simulink model "commander"  (R2021a)
settings: Solver=FixedStepAuto  StartTime=0.0  StopTime=5  FixedStep=0.02  RelTol=1e-3
(part 2 of 2)

== stateflow chart commander/Commander ==
  state initialize [parallel]
    en:
    % 初始化结构体（全局变量结尾加下划线）
    vehicle_status_out_ = px4_vehicle_status_zero();
    led_control_out_ = px4_led_control_zero();
    armed_out_ = px4_actuator_armed_zero();
    home_position_out_ = px4_home_position_zero();
    vehicle_status_flags_out_ = px4_vehicle_status_flags_zero();
    land_detector_ = land_detector;
    battery_status_out_ = px4_battery_status_zero();
    internal_state_out_ = px4_commander_state_zero();
    % 初始化相关的结构体成员变量
    land_detector_.landed = true;
    % XXX for now just set sensors as initialized
    vehicle_status_flags_out_.condition_system_sensors_initialized = true;
    % We want to accept RC inputs as default
    vehicle_status_out_.rc_input_mode = uint8(PX4_VEHICLE_STATUS.RC_IN_MODE_DEFAULT);
    vehicle_status_out_.nav_state = uint8(PX4_VEHICLE_STATUS.NAVIGATION_STATE_MANUAL);
    vehicle_status_out_.nav_state_timestamp = uint64(getSimulationTime * 1e+6);
    vehicle_status_out_.arming_state = uint8(PX4_VEHICLE_STATUS.ARMING_STATE_INIT);
    % mark all signals lost as long as they haven't been found
    vehicle_status_out_.rc_signal_lost = true;
    vehicle_status_out_.data_link_lost = true;
    % vehicle_status_flags
    vehicle_status_flags_out_.offboard_control_signal_lost = true;
    vehicle_status_flags_out_.condition_power_input_valid = true;
    vehicle_status_flags_out_.rc_calibration_valid = true;
    % default for vtol is rotary wing
    vtol_status_.vtol_in_rw_mode = true;
    % LED和蜂鸣器初始化
    led_init();
    buzzer_init();
    % 参数更新
    get_circuit_breaker_params();
    % 更新载具类型
    update_vehicle_status();
    % 记录commander启动时间
    boot_timestamp_ = uint64(getSimulationTime * 1e+6);
    % 初始化相关时间
    last_lpos_fail_time_us_ = boot_timestamp_;
    last_gpos_fail_time_us_ = boot_timestamp_;
    last_lvel_fail_time_us_ = boot_timestamp_;
    % 解锁方式
    arm_auth_init();
    settings: executionOrder=1
  state topic_update [parallel]
    settings: executionOrder=2
    state parameters_update [parallel]
      en,du:
      % 是否使能避障
      vehicle_status_flags_out_.avoidance_system_required = boolean(COM_OBS_AVOID);
      % 参数更新
      if (hasChanged(params_update.timestamp) || param_init_forced_)
      % updateParams();
      % 未解锁状态下才能修改的参数
      if(~actuator_armed.armed)
      is_rotary = is_rotary_wing(vehicle_status_out_) || (is_vtol(vehicle_status_out_) && vtol_status.vtol_in_rw_mode);
      is_fixed = is_fixed_wing(vehicle_status_out_) ||  (is_vtol(vehicle_status_out_) && ~vtol_status.vtol_in_rw_mode);
      is_ground = is_ground_rover(vehicle_status_out_);
      end
      % 飞机模式优先级高于手动
      if (is_rotary)
      vehicle_status_out_.vehicle_type = uint8(PX4_VEHICLE_STATUS.VEHICLE_TYPE_ROTARY_WING);
      elseif (is_fixed)
      vehicle_status_out_.vehicle_type = uint8(PX4_VEHICLE_STATUS.VEHICLE_TYPE_FIXED_WING);
      elseif (is_ground)
      vehicle_status_out_.vehicle_type = uint8(PX4_VEHICLE_STATUS.VEHICLE_TYPE_ROVER);
      end
      vehicle_status_out_.is_vtol = is_vtol(vehicle_status_out_);
      vehicle_status_out_.is_vtol_tailsitter = is_vtol_tailsitter(vehicle_status_out_);
      % check and update system / component ID
      vehicle_status_out_.system_id = MAV_SYS_ID;
      vehicle_status_out_.component_id = MAV_COMP_ID;
      initialize.get_circuit_breaker_params();
      status_changed_ = true;
      % 不受解锁状态影响就可以修改的参数
      vehicle_status_flags_out_.avoidance_system_required = boolean(COM_OBS_AVOID);
      vehicle_status_out_.rc_input_mode = uint8(COM_RC_IN_MODE);
      % 解锁条件
      arm_requirements_.arm_authorization = boolean(COM_ARM_AUTH_REQ);
      arm_requirements_.esc_check = boolean(COM_ARM_CHK_ESCS);
      arm_requirements_.global_position = ~COM_ARM_WO_GPS;
      arm_requirements_.mission = boolean(COM_ARM_MIS_REQ);
      arm_requirements_.geofence = (GF_ACTION > PX4_GEOFENCE_RESULT.GF_ACTION_NONE);
      % 飞行模式槽
      flight_mode_slots_(1) = COM_FLTMODE1;
      flight_mode_slots_(2) = COM_FLTMODE2;
      flight_mode_slots_(3) = COM_FLTMODE3;
      flight_mode_slots_(4) = COM_FLTMODE4;
      flight_mode_slots_(5) = COM_FLTMODE5;
      flight_mode_slots_(6) = COM_FLTMODE6;
      % 检查airmode：yaw airmode需要使用解锁开关
      if ((MC_AIRMODE~= PARAM_INVALID) && (RC_MAP_ARM_SW ~= PARAM_INVALID))
      if (MC_AIRMODE == 2) && (RC_MAP_ARM_SW == 0)
      % airmode = 1; % change to roll/pitch airmode
      % param_set(param_airmode, &airmode);
      sprintf("Yaw Airmode requires the use of an Arm Switch")
      end
      param_init_forced_ = false;
      end
      end
      settings: executionOrder=1
    state offboard_control [parallel]
      en,du:
      % 预留
      settings: executionOrder=2
    state power_update [parallel]
      settings: executionOrder=3
      (default) -> (junction 288)
      power_update -> (junction 288) : [hasChanged(system_power.timestamp) && ...
          | (uint64(getSimulationTime * 1e+6) - system_power.timestamp) < 1e+6]
      (junction 288) -> (junction 289) [order 1] : [system_power.servo_valid && ...
          | ~system_power.brick_valid && ...
          | ~system_power.usb_connected]
      (junction 288) -> (junction 290) [order 2] : {vehicle_status_flags_out_.condition_power_input_valid = true;}
      (junction 289) -> (junction 291) : % 在只有舵机电源有效的情况下飞行，这是不安全的
          | {vehicle_status_flags_out_.condition_power_input_valid = false;}
      (junction 291) -> (junction 290)
      (junction 290) -> (junction 292)
    state land_detector_auto_disarm_update [parallel]
      en,du:
      if (hasChanged(land_detector.timestamp) && actuator_armed.armed)
      if ( ~home_position.manual_home && ...
      (should_set_home_on_takeoff_ == true) && land_detector_.landed && ...
      (uint64(getSimulationTime * 1e+6) > INAIR_RESTART_HOLDOFF_INTERVAL))
      if (was_landed)
      should_set_home_on_takeoff_ = ~set_home_position();
      elseif (COM_HOME_IN_AIR)
      should_set_home_on_takeoff_ = ~set_in_air_home_position();
      end
      end
      end
      % Auto disarm after 5 seconds if kill switch is engaged
      if (actuator_armed.armed && (actuator_armed.manual_lockdown || actuator_armed.lockdown))
      if (elapsed(sec) > COM_KILL_DISARM && actuator_armed.manual_lockdown)
      send(EVT_KILL_SWITCH, arming_state_transition);
      elseif (elapsed(sec) > COM_KILL_DISARM)
      send(EVT_LOCKDOWN, arming_state_transition);
      end
      end
      settings: executionOrder=4
      state land
        en:
        if (uint64(getSimulationTime) ~= 0)
        sprintf("mavlink_log_info: Landing detected")
        end
        vehicle_status_out_.takeoff_time = uint64(0);
        was_landed = land_detector.landed;
        du:
        % 在地面期间，有以下两种情况会自动上锁
        % situation1. 着陆后，经过COM_DISARM_LAND秒后，无人机自动上锁；
        % situation2. 解锁后，COM_DISARM_PRFLT秒内不起飞，无人机自动上锁；
        state situation1 [parallel]
          en,du:
          if (have_taken_off_since_arming && COM_DISARM_LAND > 0)
          if (elapsed(sec) > COM_DISARM_LAND)
          send(EVT_AUTO_DISARM_LAND, arming_state_transition);
          end
          end
          settings: executionOrder=1
        state situation2 [parallel]
          en,du:
          if (~have_taken_off_since_arming && COM_DISARM_PRFLT > 0)
          if (elapsed(sec) > COM_DISARM_PRFLT)
          send(EVT_AUTO_DISARM_PREFLIGHT, arming_state_transition);
          end
          end
          settings: executionOrder=2
      state takeoff
        en:
        sprintf("mavlink_log_info: Takeoff detected")
        vehicle_status_out_.takeoff_time = uint64(getSimulationTime * 1e+6);
        have_taken_off_since_arming = true;
        was_landed = land_detector.landed;
        gpos_probation_time_us_ = COM_POS_FS_PROB * 1e+6;
        lpos_probation_time_us_ = gpos_probation_time_us_;
        lvel_probation_time_us_ = gpos_probation_time_us_;
      (default) -> land
      land -> takeoff : [was_landed && ...
          | ~land_detector.landed && ...
          | actuator_armed.armed]
      takeoff -> land : [~was_landed && ...
          | land_detector.landed && ...
          | actuator_armed.armed]
    state safety_update [parallel]
      en,du:
      if (hasChanged(safety_switch.timestamp))
      set_health_flags(SUBSYSTEM_TYPE_MOTORCONTROL, safety_switch.safety_switch_available, ...
      safety_switch.safety_off, safety_switch.safety_switch_available, vehicle_status_out_);
      end
      safety_disarm_allowed = (vehicle_status_out_.hil_state == uint8(PX4_VEHICLE_STATUS .HIL_STATE_OFF));
      settings: executionOrder=5
      state safety_off
        en:
        status_changed_ = true;
        if (uint64(getSimulationTime * 1e+6) ~= uint64(0))
        % set_tune(tune_control_s::TUNE_ID_NOTIFY_POSITIVE);
        end
      note: 1. 没有解锁，安全开关没有按下去的时候，不允许解锁；
          | 2. 已经解锁，安全开关按下去，则加锁；
      state safety_on
        en:
        status_changed_ = true;
        % 闪烁白色LED，蜂鸣器neutral音调
        % tune_neutral(true);
        en,du:
        % 在着陆的状态下，才允许上锁
        if (actuator_armed.armed && land_detector.landed)
        send(EVT_DISARM, arming_state_transition);
        end
      (default) -> safety_off
      safety_off -> safety_on : [hasChanged(safety_switch.timestamp) && ...
          | safety_switch.safety_switch_available && ...
          | ~safety_switch.safety_off]
      safety_on -> safety_off : [hasChanged(safety_switch.timestamp) && ...
          | safety_switch.safety_switch_available && ...
          | safety_switch.safety_off]
    state mission_result_update [parallel]
      en:
      % start mission result check
      if (hasChanged(mission_result.timestamp))
      evaluate_mission_state();
      end
      % Transition main state to loiter or auto-mission after takeoff is completed.
      if (actuator_armed.armed && ~land_detector.landed && ...
      (vehicle_status_out_.nav_state == uint8(PX4_VEHICLE_STATUS.NAVIGATION_STATE_AUTO_TAKEOFF)) && ...
      (mission_result.timestamp >= vehicle_status_out_.nav_state_timestamp) && ...
      mission_result.finished)
      if (COM_TAKEOFF_ACT == 1  && vehicle_status_flags_out_.condition_auto_mission_available)
      main_state_transition(PX4_COMMANDER_STATE.MAIN_STATE_AUTO_MISSION);
      else
      main_state_transition(PX4_COMMANDER_STATE.MAIN_STATE_AUTO_LOITER);
      end
      end
      settings: executionOrder=10
    state vtol_vehicle_status_update [parallel]
      en,du:
      % update vtol vehicle status
      if (hasChanged(vtol_status.timestamp))
      % vtol status changed
      vehicle_status_out_.vtol_fw_permanent_stab = vtol_status.fw_permanent_stab;
      % Make sure that this is only adjusted if vehicle really is of type vtol
      if (is_vtol(vehicle_status_out_))
      % Check if there has been any change while updating the flags
      if (vtol_status.vtol_in_rw_mode) % 转换和多旋翼阶段
      new_vehicle_type = uint8(PX4_VEHICLE_STATUS.VEHICLE_TYPE_ROTARY_WING);
      else  % 纯固定翼
      new_vehicle_type = uint8(PX4_VEHICLE_STATUS.VEHICLE_TYPE_FIXED_WING);
      end
      if (new_vehicle_type ~= vehicle_status_out_.vehicle_type)
      % 根据vtol_status确定飞机处于哪个阶段
      vehicle_status_out_.vehicle_type = new_vehicle_type;
      status_changed_ = true;
      end
      if (vehicle_status_out_.in_transition_mode ~= vtol_status.vtol_in_trans_mode)
      vehicle_status_out_.in_transition_mode = vtol_status.vtol_in_trans_mode;
      status_changed_ = true;
      end
      if (vehicle_status_out_.in_transition_to_fw ~= vtol_status.in_transition_to_fw)
      vehicle_status_out_.in_transition_to_fw = vtol_status.in_transition_to_fw;
      status_changed_ = true;
      end
      if (vehicle_status_flags_out_.vtol_transition_failure ~= vtol_status.vtol_transition_failsafe)
      vehicle_status_flags_out_.vtol_transition_failure = vtol_status.vtol_transition_failsafe;
      status_changed_ = true;
      end
      % 旋翼阶段取消电调的限幅
      should_soft_stop = (vehicle_status_out_.vehicle_type ~= uint8(PX4_VEHICLE_STATUS.VEHICLE_TYPE_ROTARY_WING));
      if (actuator_armed.soft_stop ~= should_soft_stop)
      armed_out_.soft_stop = should_soft_stop;
      status_changed_ = true;
      end
      end
      end
      settings: executionOrder=6
    state esc_status_update [parallel]
      en,du:
      % 预留
      settings: executionOrder=7
    state estimator_check [parallel]
      en,du:
      % 预留
      settings: executionOrder=8
    state battery_status_check [parallel]
      en,du:
      [battery_warning, battery_warning_level_increased_while_armed] = battery_check();
      settings: executionOrder=9
      (default) -> (junction 657) : % execute battery failsafe if the state has gotten worse while we are armed
      battery_status_check -> (junction 657) : [battery_warning_level_increased_while_armed]
      (junction 657) -> (junction 658) [order 1] : [battery_warning == uint8(PX4_BATTERY_STATUS.BATTERY_WARNING_NONE)]
      (junction 657) -> (junction 659) [order 2]
      (junction 658) -> (junction 666)
      (junction 659) -> (junction 660) [order 1] : [battery_warning == uint8(PX4_BATTERY_STATUS.BATTERY_WARNING_LOW)]
      (junction 659) -> (junction 661) [order 2]
      (junction 660) -> (junction 665) : {sprintf("mavlink_log_critical, Low battery level! Return advised")}
      (junction 661) -> (junction 662) [order 1] : [battery_warning == uint8(PX4_BATTERY_STATUS.BATTERY_WARNING_CRITICAL)]
      (junction 661) -> (junction 663) [order 2]
      (junction 662) -> (junction 664) : {battery_warning_critical();}
      (junction 663) -> (junction 672) [order 1] : [battery_warning == uint8(PX4_BATTERY_STATUS.BATTERY_WARNING_EMERGENCY)]
      (junction 663) -> (junction 667) [order 2]
      (junction 672) -> (junction 680) : {battery_warning_emergency();}
      (junction 667) -> (junction 678) [order 1] : [battery_warning == uint8(PX4_BATTERY_STATUS.BATTERY_WARNING_FAILED)]
      (junction 667) -> (junction 674) [order 2]
      (junction 678) -> (junction 681) : {sprintf("mavlink_log_emergency, Battery failure detected")}
      (junction 681) -> (junction 674)
      (junction 680) -> (junction 681)
      (junction 664) -> (junction 680)
      (junction 665) -> (junction 664)
      (junction 666) -> (junction 665)
      (junction 674) -> (junction 675)
    state geofence_update [parallel]
      % 预留
      settings: executionOrder=11
    state manual_control_input_handling [parallel]
      settings: executionOrder=13
    state data_link_check [parallel] [commented out]
    state avoidance_check [parallel] [commented out]
    state check_mission_flight_termination [parallel]
      en,du:
      if (actuator_armed.armed && mission_result.flight_termination && ...
      ~vehicle_status_flags_out_.circuit_breaker_flight_termination_disabled)
      armed_out_.force_failsafe = true;
      status_changed_ = true;
      sprintf("mavlink_log_critical, Geofence violation! Flight terminated")
      end
      settings: executionOrder=12
    state actuator_control_update [parallel] [commented out]
    state failure_detector_update [parallel] [commented out]
    state home_position_update [parallel] [commented out]
    state check_arming_state_change [parallel] [commented out]
    state publish_topic [parallel] [commented out]
  note: disarm() + armed()
      | arming_state_transition
  note: 存储armed状态有
      | （1）_status.arming_state（上一拍state）
      | （2）_armed.armed（true,false）
  state arming_state_transition [parallel]
    en,du:
    hil_enabled = (vehicle_status_out_.hil_state == PX4_VEHICLE_STATUS.HIL_STATE_ON);
    settings: executionOrder=3
    state init_precheck
      en:
    state standby_error [commented out]
      en:
    state standby_disarm
      state hil_enable [parallel]
        en:
        if (hil_enabled)
        status_changed_ = true;
        % enforce lockdown in HIL
        armed_out_.lockdown = true;
        vehicle_status_flags_out_.condition_system_sensors_initialized = true;
        % recover from a prearm fail
        if (vehicle_status_out_.arming_state == uint8(PX4_VEHICLE_STATUS.ARMING_STATE_STANDBY_ERROR))
        vehicle_status_out_.arming_state = uint8(PX4_VEHICLE_STATUS.ARMING_STATE_STANDBY);
        end
        % HIL can always go to standby
        % if (new_arming_state == vehicle_status_s::ARMING_STATE_STANDBY)
        % valid_transition = true;
        % end
        end
        settings: executionOrder=1
      state disarm_by_safety_button [parallel]
        en:
        if (~hil_enabled && vehicle_status_flags_out_.condition_system_sensors_initialized)
        status_changed_ = true;
        armed_out_.armed = false;
        armed_out_.ready_to_arm = true;
        vehicle_status_out_.arming_state = uint8(PX4_VEHICLE_STATUS.ARMING_STATE_STANDBY);
        vehicle_status_out_.latest_disarming_reason = uint8(PX4_ARM_DISARM_REASON.SAFETY_BUTTON);
        vehicle_status_out_.armed_time = uint64(0);
        sprintf("_mavlink_log_pub, Disarmed by safety button");
        end
        settings: executionOrder=2
      state arm_state_trans_to_standby [parallel]
        en:
        % If arming_state in INIT state, try to proceed to STANDBY state
        if (~hil_enabled && ...
        ~vehicle_status_flags_out_.condition_calibration_enabled && ...
        vehicle_status_out_.arming_state == PX4_VEHICLE_STATUS.ARMING_STATE_INIT)
        arm_state_in_init_tans_to_standby();
        end
        settings: executionOrder=3
    state armed
      en,du:
    state in_air_restore [commented out]
      en:
    state shutdown [commented out]
    init_precheck -> standby_error [commented out]
    (default) -> init_precheck
    standby_error -> init_precheck [commented out]
    standby_disarm -> standby_error [commented out]
    init_precheck -> standby_disarm : [EVT_DISARM || ...
        | ~vehicle_status_flags_out_.condition_calibration_enabled && ...
        | preflightCheck(true)]
    standby_disarm -> init_precheck [commented out] : % preflightcheck
    armed -> standby_error [commented out]
    standby_disarm -> armed : [false]
    armed -> in_air_restore [commented out]
    armed -> standby_disarm : [EVT_AUTO_DISARM_LAND || ...
        | EVT_AUTO_DISARM_PREFLIGHT]
    in_air_restore -> armed [commented out]
    standby_disarm -> shutdown [commented out] : [ ]
  state nav_state [parallel] [commented out]
  state command_long [parallel] [commented out]
    state VEHICLE_CMD_DO_REPOSITION [parallel] [commented out]
      en,du:
      if (haschanged&&cmd==xxx)
      end
  data: CBRK_BUZZER_KEY constant single =782097; CBRK_SUPPLY_CHK_KEY constant single =894281; CBRK_RATE_CTRL_KEY constant single =140253; CBRK_IO_SAFETY_KEY constant single =22027; CBRK_AIRSPD_CHK_KEY constant single =162128; CBRK_FLIGHTTERM_KEY constant single =121212; CBRK_ENGINEFAIL_KEY constant single =284953; CBRK_USB_CHK_KEY constant single =197848; CBRK_VELPOSERR_KEY constant single =201607; CBRK_VTOLARMING_KEY constant single =159753; is_rotary local boolean size=1 =false; is_fixed local boolean size=1 =false; is_ground local boolean size=1 =false; result function_output; home_pos function_input size=1; local_pos function_input size=1; gpos function_input Bus: px4_vehicle_global_position size=1; result function_output boolean size=1; home_pos function_input; lat function_input; lon function_input; alt function_input; result function_output boolean size=1; was_landed local boolean size=1 =true; INAIR_RESTART_HOLDOFF_INTERVAL constant uint64 size=1 =uint64(500); ref_pos local Bus: px4_map_projection_reference size=1; home_lat local double size=1; home_lon local double size=1; home_alt local single size=1; have_taken_off_since_arming local boolean size=1 =false; subsystem_type function_input; present function_input; enabled function_input; ok function_input; status function_input; safety_disarm_allowed local boolean size=1 =false; use_buzzer function_input; use_buzzer function_input; use_buzzer function_input; new_vehicle_type local uint8 size=1 =uint8(0); should_soft_stop local boolean size=1 =false; batt_warn function_output; batt_warn_inc_while_armed function_output; battery_warning local uint8 size=1 =uint8(0); battery_warning_level_increased_while_armed local boolean size=1 =false; batteries local Bus: px4_battery_status size=1; current_status function_input; result function_output; current_status function_input; result function_output; current_status function_input; result function_output; current_status function_input; result function_output; current_status function_input; result function_output; current_status function_input; result function_output; ret function_output; report_failures function_input; max_mandatory_gyro_count constant uint8 =uint8(1); max_optional_gyro_count constant uint8 =uint8(4); max_mandatory_accel_count constant uint8 =uint8(1); max_optional_accel_count constant uint8 =uint8(4); max_mandatory_mag_count constant uint8 =uint8(1); max_optional_mag_count constant uint8 =uint8(4); max_mandatory_baro_count constant uint8 =uint8(1); max_optional_baro_count constant uint8 =uint8(4); ret function_output; ret function_output; ret function_output; hil_enabled local boolean size=1 =false; ret function_output; ret function_output; ret function_output; ret function_output; ret function_output; ret function_output; ret function_output; ret function_output; ret function_output; ret function_output; ret function_output; ret function_output; ret function_output; ret function_output; new_main_state function_input; boot_timestamp_ local uint64 size=1 =uint64(0); last_lpos_fail_time_us_ local uint64 size=1 =uint64(0); last_gpos_fail_time_us_ local uint64 size=1 =uint64(0); last_lvel_fail_time_us_ local uint64 size=1 =uint64(0); vehicle_status_out_ output Bus: px4_vehicle_status size=1; led_control_out_ output Bus: px4_led_control size=1; tune_durations_ local uint32 size=[1 20]; CBRK_SUPPLY_CHK parameter size=1; MAV_TYPE parameter size=1; CBRK_USB_CHK parameter size=1; CBRK_AIRSPD_CHK parameter size=1; CBRK_ENGINEFAIL parameter size=1; CBRK_FLIGHTTERM parameter size=1; CBRK_VELPOSERR parameter size=1; CBRK_VTOLARMING parameter size=1; param_init_forced_ local boolean size=1 =true; VEHICLE_TYPE_FIXED_WING constant uint8 size=1 =uint8(1); VEHICLE_TYPE_QUADROTOR constant uint8 size=1 =uint8(2); VEHICLE_TYPE_COAXIAL constant uint8 size=1 =uint8(3); VEHICLE_TYPE_HELICOPTER constant uint8 size=1 =uint8(4); VEHICLE_TYPE_GROUND_ROVER constant uint8 size=1 =uint8(10); VEHICLE_TYPE_HEXAROTOR constant uint8 size=1 =uint8(13); VEHICLE_TYPE_OCTOROTOR constant uint8 size=1 =uint8(14); VEHICLE_TYPE_TRICOPTER constant uint8 size=1 =uint8(15); VEHICLE_TYPE_VTOL_DUOROTOR constant uint8 size=1 =uint8(19); VEHICLE_TYPE_VTOL_QUADROTOR constant uint8 size=1 =uint8(20); VEHICLE_TYPE_VTOL_TILTROTOR constant uint8 size=1 =uint8(21); VEHICLE_TYPE_VTOL_RESERVED2 constant uint8 size=1 =uint8(22); VEHICLE_TYPE_VTOL_RESERVED3 constant uint8 size=1 =uint8(23); VEHICLE_TYPE_VTOL_RESERVED4 constant uint8 size=1 =uint8(24); VEHICLE_TYPE_VTOL_RESERVED5 constant uint8 size=1 =uint8(25); MAV_SYS_ID parameter size=1; COM_ARM_AUTH_TO parameter size=1; param_com_arm_auth_timout_ local uint64 size=1 =uint64(0); COM_ARM_AUTH_MET parameter size=1; COM_ARM_AUTH_ID parameter size=1; params_update input Bus: px4_parameter_update size=1; actuator_armed input Bus: px4_actuator_armed size=1; vtol_status input Bus: px4_vtol_vehicle_status size=1; status_changed_ local boolean size=1 =true; MAV_COMP_ID parameter size=1; vehicle_status_flags_out_ output Bus: px4_vehicle_status_flags size=1; COM_OBS_AVOID parameter size=1; COM_RC_IN_MODE parameter size=1; arm_requirements_ local px4_arm_requqirements size=1; COM_ARM_AUTH_REQ parameter size=1; COM_ARM_CHK_ESCS parameter size=1; COM_ARM_MIS_REQ parameter size=1; GF_ACTION parameter size=1; flight_mode_slots_ local int32 size=[1 6]; COM_ARM_WO_GPS parameter size=1; MC_AIRMODE parameter size=1; PARAM_INVALID constant uint16 size=1 =0xffff; RC_MAP_ARM_SW parameter size=1; COM_FLTMODE1 parameter size=1; COM_FLTMODE2 parameter size=1; COM_FLTMODE3 parameter size=1; COM_FLTMODE4 parameter size=1; COM_FLTMODE5 parameter size=1; COM_FLTMODE6 parameter size=1; system_power input Bus: px4_system_power size=1; land_detector input Bus: px4_vehicle_land_detected size=1; COM_POS_FS_PROB parameter size=1; gpos_probation_time_us_ local uint64 size=1 =uint64(0); lpos_probation_time_us_ local uint64 size=1 =uint64(0); lvel_probation_time_us_ local uint64 size=1 =uint64(0); home_position input Bus: px4_home_position size=1; should_set_home_on_takeoff_ local boolean size=1 =true; COM_HOME_IN_AIR parameter size=1; home_position_out_ output Bus: px4_home_position size=1; local_position input Bus: px4_vehicle_local_position size=1; global_position input Bus: px4_vehicle_global_position size=1; COM_HOME_H_T parameter size=1; COM_HOME_V_T parameter size=1; safety_switch input Bus: px4_safety size=1; SUBSYSTEM_TYPE_GYRO constant uint32 size=1 =bitshift(1,0); SUBSYSTEM_TYPE_ACC constant uint32 size=1 =bitshift(1,1); SUBSYSTEM_TYPE_MAG constant uint32 size=1 =bitshift(1,2); SUBSYSTEM_TYPE_ABSPRESSURE constant uint32 size=1 =bitshift(1,3); SUBSYSTEM_TYPE_DIFFPRESSURE constant uint32 size=1 =bitshift(1,4); SUBSYSTEM_TYPE_GPS constant uint32 size=1 =bitshift(1,5); SUBSYSTEM_TYPE_OPTICALFLOW constant uint32 size=1 =bitshift(1,6); SUBSYSTEM_TYPE_CVPOSITION constant uint32 size=1 =bitshift(1,7); SUBSYSTEM_TYPE_LASERPOSITION constant uint32 size=1 =bitshift(1,8); SUBSYSTEM_TYPE_EXTERNALGROUNDTRUTH constant uint32 size=1 =bitshift(1,9); SUBSYSTEM_TYPE_ANGULARRATECONTROL constant uint32 size=1 =bitshift(1,10); SUBSYSTEM_TYPE_ATTITUDESTABILIZATION constant uint32 size=1 =bitshift(1,11); SUBSYSTEM_TYPE_YAWPOSITION constant uint32 size=1 =bitshift(1,12); SUBSYSTEM_TYPE_ALTITUDECONTROL constant uint32 size=1 =bitshift(1,13); SUBSYSTEM_TYPE_POSITIONCONTROL constant uint32 size=1 =bitshift(1,14); SUBSYSTEM_TYPE_MOTORCONTROL constant uint32 size=1 =bitshift(1,15); SUBSYSTEM_TYPE_RCRECEIVER constant uint32 size=1 =bitshift(1,16); SUBSYSTEM_TYPE_GYRO2 constant uint32 size=1 =bitshift(1,17); SUBSYSTEM_TYPE_ACC2 constant uint32 size=1 =bitshift(1,18); SUBSYSTEM_TYPE_MAG2 constant uint32 size=1 =bitshift(1,19); SUBSYSTEM_TYPE_GEOFENCE constant uint32 size=1 =bitshift(1,20); SUBSYSTEM_TYPE_AHRS constant uint32 size=1 =bitshift(1,21); SUBSYSTEM_TYPE_TERRAIN constant uint32 size=1 =bitshift(1,22); SUBSYSTEM_TYPE_REVERSEMOTOR constant uint32 size=1 =bitshift(1,23); SUBSYSTEM_TYPE_LOGGING constant uint32 size=1 =bitshift(1,24); SUBSYSTEM_TYPE_SENSORBATTERY constant uint32 size=1 =bitshift(1,25); SUBSYSTEM_TYPE_SENSORPROXIMITY constant uint32 size=1 =bitshift(1,26); SUBSYSTEM_TYPE_SATCOM constant uint32 size=1 =bitshift(1,27); SUBSYSTEM_TYPE_PREARM_CHECK constant uint32 size=1 =bitshift(1,28); SUBSYSTEM_TYPE_OBSTACLE_AVOIDANCE constant uint32 size=1 =bitshift(1,29); armed_out_ output Bus: px4_actuator_armed size=1; status_flags input Bus: px4_vehicle_status_flags size=1; land_detector_ local Bus: px4_vehicle_land_detected size=1; vtol_status_ local Bus: px4_vtol_vehicle_status size=1; COM_DISARM_LAND parameter size=1; COM_DISARM_PRFLT parameter size=1; COM_KILL_DISARM parameter size=1; battery_status input Bus: px4_battery_status size=1; battery_status_out_ output Bus: px4_battery_status size=1; rtl_flight_time input Bus: px4_rtl_flight_time size=1; BAT_CRIT_THR parameter size=1; BAT_LOW_THR parameter size=1; COM_LOW_BAT_ACT parameter size=1; BATTERY_FAILSAFE_WARNING constant uint8 size=1 =uint8(0); BATTERY_FAILSAFE_RETURN constant uint8 size=1 =uint8(1); BATTERY_FAILSAFE_LAND constant uint8 size=1 =uint8(2); BATTERY_FAILSAFE_RETURN_OR_LAND constant uint8 size=1 =uint8(3); internal_state_out_ output Bus: px4_commander_state size=1; TRANSITION_DENIED constant int8 size=1 =int8(-1); TRANSITION_NOT_CHANGED constant int8 size=1 =int8(0); TRANSITION_CHANGED constant int8 size=1 =int8(1); SYS_HAS_MAG parameter size=1; mission_result input Bus: px4_mission_result size=1; COM_TAKEOFF_ACT parameter size=1
  events: EVT_DISARM local FUNCTION_CALL_EVENT; EVT_AUTO_DISARM_LAND local FUNCTION_CALL_EVENT; EVT_AUTO_DISARM_PREFLIGHT local FUNCTION_CALL_EVENT; EVT_KILL_SWITCH local FUNCTION_CALL_EVENT; EVT_LOCKDOWN local FUNCTION_CALL_EVENT
  function led_init:
    | function led_init()
    | 
    | blink_msg_end = 0;
    | led_control_out_.led_mask = 0xff;
    | led_control_out_.mode = uint8(PX4_LED_CONTROL.MODE_OFF);
    | led_control_out_.priority = uint8(0);
    | led_control_out_.timestamp = uint64(getSimulationTime * 1e+6);
    | 
    | % led_control_pub = orb_advertise_queue(ORB_ID(led_control), &led_control, led_control_s::ORB_QUEUE_LENGTH);
    | %
    | % /* first open normal LEDs */
    | % fd_leds = px4_open(LED0_DEVICE_PATH, O_RDWR);
    | %
    | % if (fd_leds < 0) {
    | %     // there might not be an LED available, so don't make this an error
    | %     PX4_INFO("LED: open %s failed (%i)", LED0_DEVICE_PATH, errno);
    | %     return -errno;
    | %     }
    | %
    | %     /* the green LED is only available on FMUv5 */
    | %     px4_ioctl(fd_leds, LED_ON, LED_GREEN);
    | %
    | %     /* the blue LED is only available on AeroCore but not FMUv2 */
    | %     px4_ioctl(fd_leds, LED_ON, LED_BLUE);
    | %
    | %     /* switch blue off */
    | %         led_off(LED_BLUE);
    | %
    | %         /* we consider the amber led mandatory */
    | %         if (px4_ioctl(fd_leds, LED_ON, LED_AMBER)) {
    | %             PX4_WARN("Amber LED: ioctl fail");
    | %             return PX4_ERROR;
    | %             }
    | %
    | %             /* switch amber off */
    | %                 led_off(LED_AMBER);
    | 
    | end
  function buzzer_init:
    | function buzzer_init()
    | 
    | tune_durations_(uint8(PX4_TUNE_CONTROL.TUNE_ID_NOTIFY_POSITIVE)) = 800000;
    | tune_durations_(uint8(PX4_TUNE_CONTROL.TUNE_ID_NOTIFY_NEGATIVE)) = 900000;
    | tune_durations_(uint8(PX4_TUNE_CONTROL.TUNE_ID_NOTIFY_NEUTRAL)) = 500000;
    | tune_durations_(uint8(PX4_TUNE_CONTROL.TUNE_ID_ARMING_WARNING)) = 3000000;
    | tune_durations_(uint8(PX4_TUNE_CONTROL.TUNE_ID_HOME_SET)) = 800000;
    | tune_durations_(uint8(PX4_TUNE_CONTROL.TUNE_ID_BATTERY_WARNING_FAST)) = 800000;
    | tune_durations_(uint8(PX4_TUNE_CONTROL.TUNE_ID_BATTERY_WARNING_SLOW)) = 800000;
    | tune_durations_(uint8(PX4_TUNE_CONTROL.TUNE_ID_SINGLE_BEEP)) = 300000;
    | % tune_control_pub = orb_advertise_queue(ORB_ID(tune_control), &tune_control, tune_control_s::ORB_QUEUE_LENGTH);
    | 
    | end
  function get_circuit_breaker_params:
    | function get_circuit_breaker_params()
    | 
    | status_flags_out_.circuit_breaker_engaged_power_check = (CBRK_SUPPLY_CHK == CBRK_SUPPLY_CHK_KEY);
    | status_flags_out_.circuit_breaker_engaged_usb_check = (CBRK_USB_CHK == CBRK_USB_CHK_KEY);
    | status_flags_out_.circuit_breaker_engaged_airspd_check = (CBRK_AIRSPD_CHK == CBRK_AIRSPD_CHK_KEY);
    | status_flags_out_.circuit_breaker_engaged_enginefailure_check = (CBRK_ENGINEFAIL == CBRK_ENGINEFAIL_KEY);
    | status_flags_out_.circuit_breaker_flight_termination_disabled = (CBRK_FLIGHTTERM == CBRK_FLIGHTTERM_KEY);
    | status_flags_out_.circuit_breaker_engaged_posfailure_check = (CBRK_VELPOSERR == CBRK_VELPOSERR_KEY);
    | status_flags_out_.circuit_breaker_vtol_fw_arming_check = (CBRK_VTOLARMING == CBRK_VTOLARMING_KEY);
    | 
    | end
  function update_vehicle_status:
    | function update_vehicle_status()
    | 
    | vehicle_status_out_.system_type = uint8(MAV_TYPE);
    | 
    | if (is_rotary_wing(vehicle_status_out_) || is_vtol(vehicle_status_out_))
    |     vehicle_status_out_.vehicle_type = uint8(PX4_VEHICLE_STATUS.VEHICLE_TYPE_ROTARY_WING);
    | elseif (is_fixed_wing(vehicle_status_out_))
    |     vehicle_status_out_.vehicle_type = uint8(PX4_VEHICLE_STATUS.VEHICLE_TYPE_FIXED_WING);
    | elseif (is_ground_rover(vehicle_status_out_))
    |     vehicle_status_out_.vehicle_type = uint8(PX4_VEHICLE_STATUS.VEHICLE_TYPE_ROVER);
    | else
    |     vehicle_status_out_.vehicle_type = uint8(PX4_VEHICLE_STATUS.VEHICLE_TYPE_UNKNOWN);
    | end
    | 
    | vehicle_status_out_.is_vtol = is_vtol(vehicle_status_out_);
    | vehicle_status_out_.is_vtol_tailsitter = is_vtol_tailsitter(vehicle_status_out_);
    | vehicle_status_out_.system_id = uint8(MAV_SYS_ID);
    | 
    | end
  function arm_auth_init:
    | function arm_auth_init()
    | 
    | timeout = single(0.0);
    | timeout = COM_ARM_AUTH_TO;
    | param_com_arm_auth_timout_ = uint64(timeout * 1e+6);
    | 
    | auth_method = int32(PX4_ARM_AUTH_METHODS.ARM_AUTH_METHOD_ARM_REQ);
    | auth_method = COM_ARM_AUTH_MET;
    | 
    | % 如果是两步解锁
    | if (auth_method >= 0 && auth_method < int32(PX4_ARM_AUTH_METHODS.ARM_AUTH_METHOD_LAST))
    |     param_com_arm_auth_method_ = auth_method;
    | else
    |     param_com_arm_auth_method_ = int32(PX4_ARM_AUTH_METHODS.ARM_AUTH_METHOD_ARM_REQ);
    | end
    | 
    | param_com_arm_auth_id_ = COM_ARM_AUTH_ID;
    | 
    | % system_id = status_.system_id;
    | % command_ack_sub = orb_subscribe(ORB_ID(vehicle_command_ack));
    | % mavlink_log_pub = mav_log_pub;
    | 
    | end
  function result = set_home_position:
    | function result = set_home_position()
    | 
    | % Need global and local position fix to be able to set home
    | % but already set the home position in local coordinates if available
    | % in case the global position is only valid after takeoff
    | if (vehicle_status_flags_out_.condition_local_position_valid)
    |     
    |     home_position_out_.timestamp = uint64(getSimulationTime * 1e+6);
    |     home_position_out_.manual_home = false;
    |     land_detector_auto_disarm_update.fillLocalHomePos(home_position_out_, local_position);
    |     
    |     if (vehicle_status_flags_out_.condition_global_position_valid)
    |         
    |         % Ensure that the GPS accuracy is good enough for intializing home
    |         if (land_detector_auto_disarm_update.isGPosGoodForInitializingHomePos(global_position))
    |             land_detector_auto_disarm_update.fillGlobalHomePos(home_position_out_, global_position.lat, global_position.lon, global_position.alt);
    |             land_detector_auto_disarm_update.setHomePosValid();
    |         end
    |     end
    |     
    | end
    | 
    | result = vehicle_status_flags_out_.condition_home_position_valid;
    | 
    | end
  function fillLocalHomePos(home_pos, local_pos):
    | function fillLocalHomePos(home_pos, local_pos)
    | 
    | home_pos.x = local_pos.x;
    | home_pos.y = local_pos.y;
    | home_pos.z = local_pos.z;
    | home_pos.valid_lpos = true;
    | home_pos.yaw = local_pos.heading;
    | 
    | end
  function result = isGPosGoodForInitializingHomePos(gpos):
    | function result = isGPosGoodForInitializingHomePos(gpos)
    | 
    | result = (gpos.eph <= COM_HOME_H_T) && (gpos.epv <= COM_HOME_V_T);
    | 
    | end
  function fillGlobalHomePos(home_pos, lat, lon, alt):
    | function fillGlobalHomePos(home_pos, lat, lon, alt)
    | 
    | home_pos.lat = lat;
    | home_pos.lon = lon;
    | home_pos.valid_hpos = true;
    | home_pos.alt = alt;
    | home_pos.valid_alt = true;
    | 
    | end
  function setHomePosValid:
    | function setHomePosValid()
    | 
    | % 	// play tune first time we initialize HOME
    | % 	if (!_status_flags.condition_home_position_valid) {
    | % 		tune_home_set(true);
    | % 	}
    | 
    | % mark home position as set
    | status_flags_out_.condition_home_position_valid = true;
    | 
    | end
  function result = set_in_air_home_position:
    | % 函数功能：
    | % 允许在飞机起飞后设置home点位置；
    | % 如果参数COM_HOME_IN_AIR设置为true，飞机可以在起飞后设置其home点位置；
    | % 如果一个local_pos估计是准确的，则反向计算真正的home点位置；
    | % 如果没有有效的local_pos，则将home点设置为当前位置。
    | % PARAM_DEFINE_INT32(COM_HOME_IN_AIR, 0);
    | function result = set_in_air_home_position()
    | 
    | if (vehicle_status_flags_out_.condition_local_position_valid && ...
    |         vehicle_status_flags_out_.condition_global_position_valid)
    |     
    |     % Ensure that the GPS accuracy is good enough for intializing home
    |     if (land_detector_auto_disarm_update.isGPosGoodForInitializingHomePos(global_position))
    |         
    |         home_position_out_.timestamp = uint64(getSimulationTime * 1e+6);
    |         
    |         if (home_position_out_.valid_lpos)
    |             % Back-compute lon, lat and alt of home position given the home
    |             % and current positions in local frame
    |             ref_pos = map_projection_init(global_position.lat, global_position.lon);
    |             [result, home_lat, home_lon] = map_projection_reproject(ref_pos, home_position.x - local_position.x, home_position.y - local_position.y);
    |             home_alt = single(global_position.alt + home_position.z);
    |             land_detector_auto_disarm_update.fillGlobalHomePos(home_position, home_lat, home_lon, home_alt);
    |         else
    |             % Home position in local frame is unknowm, set
    |             % home as current position
    |             land_detector_auto_disarm_update.fillLocalHomePos(home_position_out_, local_position);
    |             land_detector_auto_disarm_update.fillGlobalHomePos(home_position_out_, global_position.lon, global_position.lat, global_position.alt);
    |         end
    |         
    |         land_detector_auto_disarm_update.setHomePosValid();
    |         
    |     end
    | end
    | 
    | result = vehicle_status_flags_out_.condition_home_position_valid;
    | 
    | end
  function set_health_flags(subsystem_type, present, enabled, ok, status):
    | function set_health_flags(subsystem_type, present, enabled, ok, status)
    | 
    | sprintf("set_health_flags: Type %llu pres=%u enabl=%u ok=%u")
    | 
    | % if (present) {
    | %     status.onboard_control_sensors_present |= (uint32_t)subsystem_type;
    | % } else {
    | %     status.onboard_control_sensors_present &= ~(uint32_t)subsystem_type;
    | % }
    | % 
    | % if (enabled) {
    | %     status.onboard_control_sensors_enabled |= (uint32_t)subsystem_type;
    | % } else {
    | %     status.onboard_control_sensors_enabled &= ~(uint32_t)subsystem_type;
    | % }
    | % 
    | % if (ok) {
    | %     status.onboard_control_sensors_health |= (uint32_t)subsystem_type;
    | % } else {
    | %     status.onboard_control_sensors_health &= ~(uint32_t)subsystem_type;
    | % }
    | 
    | if (present)
    |     status.onboard_control_sensors_present = bitor(status.onboard_control_sensors_present, subsystem_type);
    | else
    |     status.onboard_control_sensors_present = bitand(status.onboard_control_sensors_present, bitcmp(subsystem_type));
    | end
    | 
    | if (enabled)
    |     status.onboard_control_sensors_enabled = bitor((status.onboard_control_sensors_enabled), subsystem_type);
    | else
    |     status.onboard_control_sensors_enabled = bitand((status.onboard_control_sensors_enabled), bitcmp(subsystem_type));
    | end
    | 
    | if (ok)
    |     status.onboard_control_sensors_health = bitor(status.onboard_control_sensors_health, subsystem_type);
    | else
    |     status.onboard_control_sensors_health = bitand(status.onboard_control_sensors_health, bitcmp(subsystem_type));
    | end
    | 
    | end
  function evaluate_mission_state:
    | function evaluate_mission_state()
    | 
    | mission_instance_count = mission_result.instance_count;
    | 
    | % if mission_result is valid for the current mission
    | mission_result_ok = (mission_result.timestamp > boot_timestamp_) && (mission_result.instance_count > 0);
    | vehicle_status_flags_out_.condition_auto_mission_available = mission_result_ok && mission_result.valid;
    | 
    | if mission_result_ok
    |     
    |     %% check mission failure
    |     if vehicle_status_out_.mission_failure ~= mission_result.failure
    |         
    |         vehicle_status_out_.mission_failure = mission_result.failure;
    |         status_changed_ = true;
    |         
    |         if vehicle_status_out_.mission_failure
    |             sprintf("mavlink_log_critical, Mission cannot be completed")
    |         end
    |         
    |     end
    |     
    |     %% Only evaluate mission state if home is set
    |     if vehicle_status_flags_out_.condition_home_position_valid && hasChanged(mission_result.instance_count)
    |         
    |         if ~vehicle_status_flags_out_.condition_auto_mission_available
    |             % the mission is invalid
    |             tune_mission_fail(true);
    |         elseif mission_result.warning
    |             % the mission has a warning
    |             tune_mission_warn(true);
    |         else
    |             % the mission is valid
    |             tune_mission_ok(true);
    |         end
    |         
    |     end
    |     
    | end
    | 
    | end
  function tune_mission_fail(use_buzzer):
    | function tune_mission_fail(use_buzzer)
    | 
    | % blink_msg_end = hrt_absolute_time() + BLINK_MSG_TIME;
    | % rgbled_set_color_and_mode(led_control_s::COLOR_RED, led_control_s::MODE_BLINK_FAST);
    | % 
    | if use_buzzer
    | %     set_tune(tune_control_s::TUNE_ID_NOTIFY_NEGATIVE);
    | end
    | 
    | end
  function tune_mission_warn(use_buzzer):
    | function tune_mission_warn(use_buzzer)
    | 
    | % blink_msg_end = hrt_absolute_time() + BLINK_MSG_TIME;
    | % rgbled_set_color_and_mode(led_control_s::COLOR_YELLOW, led_control_s::MODE_BLINK_FAST);
    | % 
    | if use_buzzer
    | %     set_tune(tune_control_s::TUNE_ID_NOTIFY_NEUTRAL);
    | end
    | 
    | end
  function tune_mission_ok(use_buzzer):
    | function tune_mission_ok(use_buzzer)
    | 
    | % blink_msg_end = hrt_absolute_time() + BLINK_MSG_TIME;
    | % rgbled_set_color_and_mode(led_control_s::COLOR_GREEN, led_control_s::MODE_BLINK_FAST);
    | % 
    | if use_buzzer
    | %     set_tune(tune_control_s::TUNE_ID_NOTIFY_POSITIVE);
    | end
    | 
    | end
  function [batt_warn, batt_warn_inc_while_armed] = battery_check:
    | function [batt_warn, batt_warn_inc_while_armed] = battery_check()
    | 
    | batt_warn = uint8(0);
    | batt_warn_inc_while_armed = false;
    | 
    | if (hasChanged(battery_status.timestamp))
    |     
    |     % 此处假定有1块电池connected
    |     num_connected_batteries = 1;
    |     
    |     % 假定所有的电池全为一样的，batteries此处设置为1块电池
    |     for (i = 1:num_connected_batteries)
    |         batteries(i) = battery_status;
    |     end
    |     
    |     worst_warning = uint8(PX4_BATTERY_STATUS.BATTERY_WARNING_NONE);
    |     oldest_update = uint64(getSimulationTime * 1e+6);
    |     
    |     battery_current = single(0.0);
    |     battery_level = single(0.0);
    |     
    |     % Only iterate over connected batteries. We don't care if a disconnected battery is not regularly publishing.
    |     for (i = 1 : num_connected_batteries)
    |         if (batteries(i).warning > worst_warning)
    |             worst_warning = batteries(i).warning;
    |         end
    |         
    |         current_time_us = uint64(getSimulationTime * 1e+6);
    |         if ((current_time_us - batteries(i).timestamp) > (current_time_us - oldest_update))
    |             oldest_update = batteries(i).timestamp;
    |         end
    |         
    |         % Sum up current from all batteries.
    |         battery_current = battery_current + batteries(i).current_filtered_a;
    |         
    |         % average levels from all batteries
    |         battery_level = battery_level + batteries(i).remaining;
    |     end
    |     
    |     battery_level = battery_level / num_connected_batteries;
    |     battery_usage_to_home = single(0.0);
    |     
    |     if (uint64(getSimulationTime * 1e+6) - rtl_flight_time.timestamp < 2*1e+6)
    |         battery_usage_to_home = rtl_flight_time.rtl_limit_fraction;
    |     end
    |     
    |     battery_range_warning = uint8(PX4_BATTERY_STATUS.BATTERY_WARNING_NONE);
    |     if (isfinite(battery_usage_to_home))
    |         
    |         battery_at_home = battery_level - battery_usage_to_home;
    |         if (battery_at_home < BAT_CRIT_THR)
    |             battery_range_warning = uint8(PX4_BATTERY_STATUS.BATTERY_WARNING_CRITICAL);
    |         elseif (battery_at_home < BAT_LOW_THR)
    |             battery_range_warning = uint8(PX4_BATTERY_STATUS.BATTERY_WARNING_LOW);
    |         end
    |         
    |         if (battery_range_warning > worst_warning)
    |             worst_warning = battery_range_warning;
    |         end
    |         
    |         batt_warn_inc_while_armed = false;
    |         update_internal_battery_state = false;
    |         
    |         if (actuator_armed.armed)
    |             if (worst_warning > batt_warn)
    |                 batt_warn_inc_while_armed = true;
    |                 update_internal_battery_state = true;
    |             elseif (battery_warning ~= worst_warning)
    |                 update_internal_battery_state = true;
    |             end
    |         end
    |         
    |         if (update_internal_battery_state)
    |             batt_warn = worst_warning;
    |         end
    |         
    |         % All connected batteries are regularly being published
    |         % There is at least one connected battery (in any slot)
    |         % No currently-connected batteries have any warning
    |         vehicle_status_flags_out_.condition_battery_healthy = (uint64(getSimulationTime * 1e+6) - oldest_update < 5 * 1e+6) && ...
    |             (num_connected_batteries > 0) && (batt_warn == uint8(PX4_BATTERY_STATUS.BATTERY_WARNING_NONE));
    |     end
    |     
    | end  % function end
  function battery_warning_critical:
    | function battery_warning_critical()
    | 
    | % switch low battery action
    | switch (COM_LOW_BAT_ACT)
    |     
    |     case BATTERY_FAILSAFE_WARNING
    |         sprintf("mavlink_log_critical, Critical battery level! landing advised")
    |         
    |     case BATTERY_FAILSAFE_RETURN || BATTERY_FAILSAFE_RETURN_OR_LAND
    |         if (status_flags.condition_global_position_valid && status_flags.condition_home_position_valid)
    |             if (~(internal_state_out_.main_state == uint8(PX4_COMMANDER_STATE.MAIN_STATE_AUTO_RTL) || ...
    |                     internal_state_out_.main_state == uint8(PX4_COMMANDER_STATE.MAIN_STATE_AUTO_LAND) || ...
    |                     internal_state_out_.main_state == uint8(PX4_COMMANDER_STATE.MAIN_STATE_AUTO_PRECLAND)))
    |                 internal_state_out_.main_state = uint8(PX4_COMMANDER_STATE.MAIN_STATE_AUTO_RTL);
    |                 internal_state_out_.timestamp = uint64(getSimulationTime * 1e+6);
    |                 sprintf("mavlink_log_critical, Critical battery level! executing RTL")
    |             end
    |         else
    |             if (~(internal_state_out_.main_state == uint8(PX4_COMMANDER_STATE.MAIN_STATE_AUTO_LAND) || ...
    |                     internal_state_out_.main_state == uint8(PX4_COMMANDER_STATE.MAIN_STATE_AUTO_PRECLAND)))
    |                 internal_state_out_.main_state = uint8(PX4_COMMANDER_STATE.MAIN_STATE_AUTO_LAND);
    |                 internal_state_out_.timestamp = uint64(getSimulationTime * 1e+6);
    |                 sprintf("mavlink_log_emergency, Critical battery level! can't execute RTL, landing instead")
    |             end
    |         end
    |         
    |     case BATTERY_FAILSAFE_LAND
    |         if (~(internal_state_out_.main_state == uint8(PX4_COMMANDER_STATE.MAIN_STATE_AUTO_LAND) || ...
    |                 internal_state_out_.main_state == uint8(PX4_COMMANDER_STATE.MAIN_STATE_AUTO_PRECLAND)))
    |             internal_state_out_.main_state = uint8(PX4_COMMANDER_STATE.MAIN_STATE_AUTO_LAND);
    |             internal_state_out_.timestamp = uint64(getSimulationTime * 1e+6);
    |             sprintf("mavlink_log_emergency, Critical battery level! landing")
    |         end
    |         
    | end
    | 
    | end % function end
  function battery_warning_emergency:
    | function battery_warning_emergency()
    | 
    | switch (COM_LOW_BAT_ACT)
    |     
    |     case BATTERY_FAILSAFE_WARNING
    |         sprintf("mavlink_log_emergency, Dangerous battery level! please land!")
    |         
    |     case BATTERY_FAILSAFE_RETURN
    |         if (vehicle_status_flags_out_.condition_global_position_valid && status_flags.condition_home_position_valid)
    |             if (~(internal_state_out_.main_state == uint8(PX4_COMMANDER_STATE.MAIN_STATE_AUTO_RTL) || ...
    |                     internal_state_out_.main_state == uint8(PX4_COMMANDER_STATE.MAIN_STATE_AUTO_LAND) || ...
    |                     internal_state_out_.main_state == uint8(PX4_COMMANDER_STATE.MAIN_STATE_AUTO_PRECLAND)))
    |                 internal_state_out_.main_state = uint8(PX4_COMMANDER_STATE.MAIN_STATE_AUTO_RTL);
    |                 internal_state_out_.timestamp = uint64(getSimulationTime * 1e+6);
    |                 sprintf("mavlink_log_critical, Dangerous battery level! executing RTL")
    |             elseif (~(internal_state_out_.main_state == uint8(PX4_COMMANDER_STATE.MAIN_STATE_AUTO_LAND) || ...
    |                     internal_state_out_.main_state == uint8(PX4_COMMANDER_STATE.MAIN_STATE_AUTO_PRECLAND)))
    |                 internal_state_out_.main_state = uint8(PX4_COMMANDER_STATE.MAIN_STATE_AUTO_LAND);
    |                 internal_state_out_.timestamp = uint64(getSimulationTime * 1e+6);
    |                 sprintf("mavlink_log_emergency, Dangerous battery level! can't execute RTL, landing instead")
    |             end
    |         end
    |         
    |     case BATTERY_FAILSAFE_RETURN_OR_LAND || BATTERY_FAILSAFE_LAND
    |         if (~(internal_state_out_.main_state == uint8(PX4_COMMANDER_STATE.MAIN_STATE_AUTO_LAND) || ...
    |                 internal_state_out_.main_state == uint8(PX4_COMMANDER_STATE.MAIN_STATE_AUTO_PRECLAND)))
    |             internal_state_out_.main_state = uint8(PX4_COMMANDER_STATE.MAIN_STATE_AUTO_LAND);
    |             internal_state_out_.timestamp = uint64(getSimulationTime * 1e+6);
    |             sprintf("mavlink_log_emergency, Dangerous battery level! landing");
    |         end
    | end
    | 
    | end
  function result = is_vtol_tailsitter(current_status):
    | function result = is_vtol_tailsitter(current_status)
    | 
    | result = (current_status.system_type == VEHICLE_TYPE_VTOL_DUOROTOR || ...
    |     current_status.system_type == VEHICLE_TYPE_VTOL_QUADROTOR);
    | 
    | end
  function result = is_rotary_wing(current_status):
    | function result = is_rotary_wing(current_status)
    | 
    | result = is_multirotor(current_status) || ...
    |     (current_status.system_type == VEHICLE_TYPE_HELICOPTER) || ...
    |     (current_status.system_type == VEHICLE_TYPE_COAXIAL);
    | 
    | end
  function result = is_multirotor(current_status):
    | function result = is_multirotor(current_status)
    | 
    | result = ((current_status.system_type == VEHICLE_TYPE_QUADROTOR) || ...
    |     (current_status.system_type == VEHICLE_TYPE_HEXAROTOR) || ...
    |     (current_status.system_type == VEHICLE_TYPE_OCTOROTOR) || ...
    |     (current_status.system_type == VEHICLE_TYPE_TRICOPTER));
    | 
    | end
  function result = is_ground_rover(current_status):
    | function result = is_ground_rover(current_status)
    | 
    | result = current_status.system_type == VEHICLE_TYPE_GROUND_ROVER;
    | 
    | end
  function result = is_fixed_wing(current_status):
    | function result = is_fixed_wing(current_status)
    | 
    | result = current_status.system_type == VEHICLE_TYPE_FIXED_WING;
    | 
    | end
  function result = is_vtol(current_status):
    | function result = is_vtol(current_status)
    | 
    | result = (current_status.system_type == VEHICLE_TYPE_VTOL_DUOROTOR || ...
    |     current_status.system_type == VEHICLE_TYPE_VTOL_QUADROTOR || ...
    |     current_status.system_type == VEHICLE_TYPE_VTOL_TILTROTOR || ...
    |     current_status.system_type == VEHICLE_TYPE_VTOL_RESERVED2 || ...
    |     current_status.system_type == VEHICLE_TYPE_VTOL_RESERVED3 || ...
    |     current_status.system_type == VEHICLE_TYPE_VTOL_RESERVED4 || ...
    |     current_status.system_type == VEHICLE_TYPE_VTOL_RESERVED5);
    | 
    | end
  function ret = preflightCheck(report_failures):
    | % 函数返回值(ret):
    | % TRANSITION_DENIED = -1,
    | % TRANSITION_NOT_CHANGED = 0,
    | % TRANSITION_CHANGED = 1;
    | function ret = preflightCheck(report_failures)
    | 
    | % init return value
    | ret = TRANSITION_CHANGED;
    | 
    | failed = false;
    | 
    | report_failures = (report_failures && vehicle_status_flags_out_.condition_system_hotplug_timeout && ...
    |     ~vehicle_status_flags_out_.condition_calibration_enabled);
    | 
    | failed = failed || ~airframeCheck();
    | failed = failed || ~sdcardCheck();
    | 
    | %% check mag
    | if (SYS_HAS_MAG == 1)
    |     % check all sensors individually, but fail only for mandatory ones
    |     for i = 1:max_optional_mag_count
    |         magnetometerCheck();
    |         magConsistencyCheck();
    |     end
    |     
    |     %% check accel
    |     % check all sensors individually, but fail only for mandatory ones
    |     for i = 1:max_optional_accel_count
    |         accelerometerCheck();
    |     end
    |     
    |     %% check gyro
    |     % check all sensors individually, but fail only for mandatory ones
    |     for i = 1:max_optional_gyro_count
    |         gyroCheck();
    |     end
    |     
    |     %% baro check
    |     % check all sensors individually, but fail only for mandatory ones
    |     for i = 1:max_optional_baro_count
    |         baroCheck();
    |     end
    |     
    |     %% check imu consistency
    |     % To be performed after the individual sensor checks have completed
    |     if ~imuConsistencyCheck()
    |         failed = true;
    |     end
    |     
    |     %% check airspeed
    |     if ~vehicle_status_flags_out_.circuit_breaker_engaged_airspd_check && ...
    |             (vehicle_status_out_.vehicle_type == PX4_VEHICLE_STATUS.VEHICLE_TYPE_FIXED_WING || vehicle_status_out_.is_vtol)
    |         if ~airspeedCheck()
    |             failed = true;
    |         end
    |     end
    |     
    |     %% check RC calibration
    |     rcCalibrationCheck();
    |     
    |     %% check system error
    |     powerCheck();
    |     
    |     %% check Navigation EKF
    |     ekf2Check();
    |     ekf2CheckSensorBias();
    |     
    |     %% check Failure Detector
    |     failureDetectorCheck();
    |     failed = failed || ~manualControlCheck();
    |     failed = failed || ~cpuResourceCheck();
    |     
    |     %% Report status
    |     ret = int8(~failed);
    |     
    | end
  function ret = airframeCheck:
    | function ret = airframeCheck()
    | 
    | ret = true; % success
    | 
    | end
  function ret = sdcardCheck:
    | function ret = sdcardCheck()
    | 
    | ret = true; % success
    | 
    | end
  function ret = magnetometerCheck:
    | function ret = magnetometerCheck()
    | 
    | ret = true; % success
    | 
    | end
  function arm_state_in_init_tans_to_standby:
    | function arm_state_in_init_tans_to_standby()
    | 
    | persistent last_preflight_check;
    | last_preflight_check = uint64(0);
    | 
    | if (vehicle_status_flags_out_.condition_system_sensors_initialized && ...
    |         (last_preflight_check == 0 || (uint64(getSimulationTime * 1e+6) - last_preflight_check > 1e+6)))
    |     
    | %     vehicle_status_flags_out_.condition_system_sensors_initialized = PreFlightCheck::preflightCheck(mavlink_log_pub, status,
    | %     status_flags, false, status.arming_state != vehicle_status_s::ARMING_STATE_ARMED,
    | %     time_since_boot);
    |     
    |     last_preflight_check = uint64(getSimulationTime * 1e+6);
    |     
    | end
    | 
    | end
  function ret = magConsistencyCheck:
    | function ret = magConsistencyCheck()
    | 
    | ret = true; % success
    | 
    | end
  function ret = accelerometerCheck:
    | function ret = accelerometerCheck()
    | 
    | ret = true; % success
    | 
    | end
  function ret = gyroCheck:
    | function ret = gyroCheck()
    | 
    | ret = true; % success
    | 
    | end
  function ret = baroCheck:
    | function ret = baroCheck()
    | 
    | ret = true; % success
    | 
    | end
  function ret = imuConsistencyCheck:
    | function ret = imuConsistencyCheck()
    | 
    | ret = true; % success
    | 
    | end
  function ret = airspeedCheck:
    | function ret = airspeedCheck()
    | 
    | ret = true; % success
    | 
    | end
  function ret = rcCalibrationCheck:
    | function ret = rcCalibrationCheck()
    | 
    | ret = true; % success
    | 
    | end
  function ret = powerCheck:
    | function ret = powerCheck()
    | 
    | ret = true; % success
    | 
    | end
  function ret = ekf2Check:
    | function ret = ekf2Check()
    | 
    | ret = true; % success
    | 
    | end
  function ret = ekf2CheckSensorBias:
    | function ret = ekf2CheckSensorBias()
    | 
    | ret = true; % success
    | 
    | end
  function ret = failureDetectorCheck:
    | function ret = failureDetectorCheck()
    | 
    | ret = true; % success
    | 
    | end
  function ret = manualControlCheck:
    | function ret = manualControlCheck()
    | 
    | ret = true; % success
    | 
    | end
  function ret = cpuResourceCheck:
    | function ret = cpuResourceCheck()
    | 
    | ret = true; % success
    | 
    | end
  function ret = main_state_transition(new_main_state):
    | function ret = main_state_transition(new_main_state)
    | 
    | % IMPORTANT: The assumption of callers of this function is that the execution of
    | % this check is essentially "free". Therefore any runtime checking in here has to be
    | % kept super lightweight. No complex logic or calls on external function should be
    | % implemented here.
    | 
    | ret = TRANSITION_DENIED;
    | 
    | % transition may be denied even if the same state is requested because conditions may have changed
    | switch (new_main_state)
    |     
    |     case {uint8(PX4_COMMANDER_STATE.MAIN_STATE_MANUAL) || ...
    |             uint8(PX4_COMMANDER_STATE.MAIN_STATE_STAB) || ...
    |             uint8(PX4_COMMANDER_STATE.MAIN_STATE_ACRO)}
    |         ret = TRANSITION_CHANGED;
    |         
    |     case uint8(PX4_COMMANDER_STATE.MAIN_STATE_ALTCTL)
    |         % need at minimum altitude estimate
    |         if vehicle_status_flags_out_.condition_local_altitude_valid || vehicle_status_flags_out_.condition_global_position_valid
    |             ret = TRANSITION_CHANGED;
    |         end
    |         
    |     case uint8(PX4_COMMANDER_STATE.MAIN_STATE_POSCTL)
    |         % need at minimum local position estimate
    |         if vehicle_status_flags_out_.condition_local_position_valid || vehicle_status_flags_out_.condition_global_position_valid
    |             ret = TRANSITION_CHANGED;
    |         end
    |         
    |     case uint8(PX4_COMMANDER_STATE.MAIN_STATE_AUTO_LOITER)
    |         % need global position estimate
    |         if vehicle_status_flags_out_.condition_global_position_valid
    |             ret = TRANSITION_CHANGED;
    |         end
    |         
    |     case {uint8(PX4_COMMANDER_STATE.MAIN_STATE_AUTO_FOLLOW_TARGET) || ...
    |             uint8(PX4_COMMANDER_STATE.MAIN_STATE_ORBIT) || ...
    |             uint8(PX4_COMMANDER_STATE.MAIN_STATE_ORBIT)}
    |         % Follow and orbit only implemented for multicopter
    |         if vehicle_status_out_.vehicle_type == PX4_VEHICLE_STATUS.VEHICLE_TYPE_ROTARY_WING
    |             ret = TRANSITION_CHANGED;
    |         end
    |         
    |     case uint8(PX4_COMMANDER_STATE.MAIN_STATE_AUTO_MISSION)
    |         % need global position, home position, and a valid mission
    |         if vehicle_status_flags_out_.condition_global_position_valid && ...
    |                 vehicle_status_flags_out_.condition_auto_mission_available
    |             ret = TRANSITION_CHANGED;
    |         end
    |         
    |     case uint8(PX4_COMMANDER_STATE.MAIN_STATE_AUTO_RTL)
    |         % need global position and home position
    |         if vehicle_status_flags_out_.condition_global_position_valid && ...
    |                 vehicle_status_flags_out_.condition_home_position_valid
    |             ret = TRANSITION_CHANGED;
    |         end
    |         
    |     case {uint8(PX4_COMMANDER_STATE.MAIN_STATE_AUTO_TAKEOFF)|| ...
    |             uint8(PX4_COMMANDER_STATE.MAIN_STATE_AUTO_LAND)}
    |         % need local position
    |         if vehicle_status_flags_out_.condition_local_position_valid
    |             ret = TRANSITION_CHANGED;
    |         end
    |         
    |     case uint8(PX4_COMMANDER_STATE.MAIN_STATE_AUTO_PRECLAND)
    |         % need local and global position, and precision land only implemented for multicopters
    |         if vehicle_status_flags_out_.condition_local_position_valid && ...
    |                 vehicle_status_flags_out_.condition_global_position_valid && ...
    |                 vehicle_status_out_.vehicle_type == PX4_VEHICLE_STATUS.VEHICLE_TYPE_ROTARY_WING
    |             ret = TRANSITION_CHANGED;
    |         end
    |         
    |     case uint8(PX4_COMMANDER_STATE.MAIN_STATE_OFFBOARD)
    |         % need offboard signal
    |         if ~vehicle_status_flags_out_.offboard_control_signal_lost
    |             ret = TRANSITION_CHANGED;
    |         end
    |         
    |     case uint8(PX4_COMMANDER_STATE.MAIN_STATE_MAX)
    |         
    | end
    | 
    | %% result
    | if ret == TRANSITION_CHANGED
    |     if internal_state_out_.main_state ~= uint8(new_main_state);
    |         internal_state_out_.main_state = uint8(new_main_state);
    |         internal_state_out_.main_state_changes = internal_state_out_.main_state_changes + 1;
    |         internal_state_out_.timestamp = uint64(getSimulationTime * 1e+6);
    |     else
    |         ret = TRANSITION_NOT_CHANGED;
    |     end
    | end
    | 
    | end
